simulink model "day5"  (R2024a)
settings: Solver=VariableStepAuto  StartTime=0.0  StopTime=20.0  RelTol=1e-3
libraries: simulink_extras x2
settings Model: Creator=tusha  LastModifiedBy=tusha

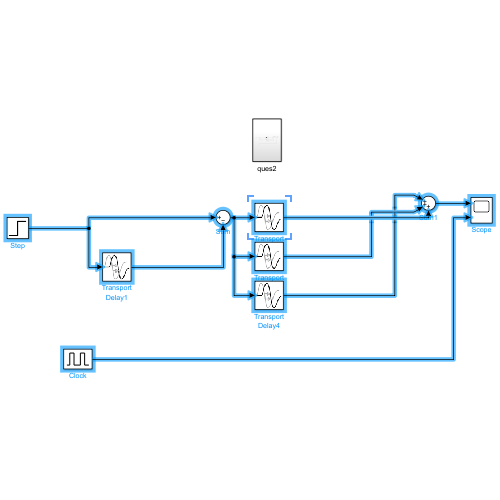
[thumbnail: Simulink's stored preview of the top-level diagram]
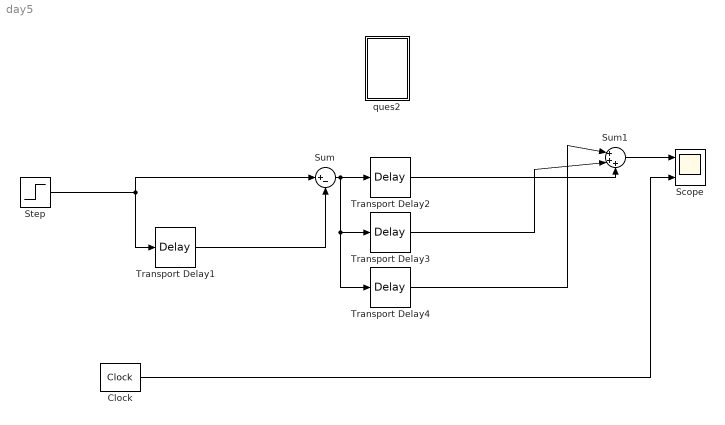
== system day5 ==
  Clock : simulink_extras/Flip Flops/Clock  period=1
  Scope : Scope  NumInputPorts=2
  Step : Step  SampleTime=0
  Sum : Sum  Inputs=|+-
  Sum1 : Sum  Inputs=|+++
  Transport Delay1 : TransportDelay
  Transport Delay2 : TransportDelay  DelayTime=11
  Transport Delay3 : TransportDelay  DelayTime=15
  Transport Delay4 : TransportDelay  DelayTime=7
  ques2 : Subsystem
  wires:
  Sum1/1 -> Scope/1
  Transport Delay1/1 -> Sum/2
  Step/1 -> Sum/1, Transport Delay1/1
  Transport Delay3/1 -> Sum1/2
  Sum/1 -> Transport Delay4/1, Transport Delay3/1, Transport Delay2/1
  Clock/1 -> Scope/2
  Transport Delay4/1 -> Sum1/1
  Transport Delay2/1 -> Sum1/3

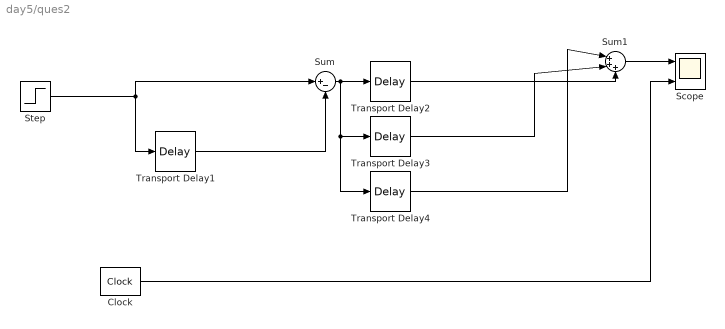
== system day5/ques2 ==
  Clock : simulink_extras/Flip Flops/Clock  period=1
  Scope : Scope  NumInputPorts=2
  Step : Step  SampleTime=0
  Sum : Sum  Inputs=|+-
  Sum1 : Sum  Inputs=|+++
  Transport Delay1 : TransportDelay
  Transport Delay2 : TransportDelay  DelayTime=11
  Transport Delay3 : TransportDelay  DelayTime=15
  Transport Delay4 : TransportDelay  DelayTime=7
  wires:
  Transport Delay4/1 -> Sum1/1
  Sum/1 -> Transport Delay4/1, Transport Delay3/1, Transport Delay2/1
  Step/1 -> Sum/1, Transport Delay1/1
  Transport Delay2/1 -> Sum1/3
  Clock/1 -> Scope/2
  Sum1/1 -> Scope/1
  Transport Delay1/1 -> Sum/2
  Transport Delay3/1 -> Sum1/2
